simulink model "VELO1"  (R2019b)
settings: Solver=FixedStepAuto  StartTime=0.0  StopTime=t(end)  FixedStep=0.01  RelTol=1e-3
libraries: eeGeneralControl x26, dspstat3 x15, dspfdesign x11, sharedTrackingLibrary x2
(part 1 of 2)
settings Model: Creator=hosseini-a  LastModifiedBy=Ali
settings OptimizationCC: DefaultParameterBehavior=Inlined  EnhancedBackFolding=on  PassReuseOutputArgsAs=Individual arguments  ZeroExternalMemoryAtStartup=off  ZeroInternalMemoryAtStartup=off  OptimizeBlockOrder=speed  DifferentSizesBufferReuse=on  OptimizationCustomize=off  EfficientTunableParamExpr=on
settings DebuggingCC: ParameterTunabilityLossMsg=error
settings SFSimCC: MATLABDynamicMemAlloc=off
settings RTWCC: SystemTargetFile=ert.tlc  TemplateMakefile=ert_default_tmf  GenerateReport=on  IncludeHyperlinkInReport=on  LaunchReport=on  GenerateTraceInfo=on  GenerateTraceReport=on  GenerateTraceReportSl=on  GenerateTraceReportSf=on  GenerateTraceReportEml=on
settings CodeAppCC: ForceParamTrailComments=on  IgnoreCustomStorageClasses=off  OperatorAnnotations=on  SimulinkDataObjDesc=on  SFDataObjDesc=on  InsertBlockDesc=on
settings ERTTargetCC: TargetLangStandard=C99 (ISO)  GenerateSampleERTMain=on  InlinedParameterPlacement=NonHierarchical  ERTCustomFileTemplate=example_file_process.tlc

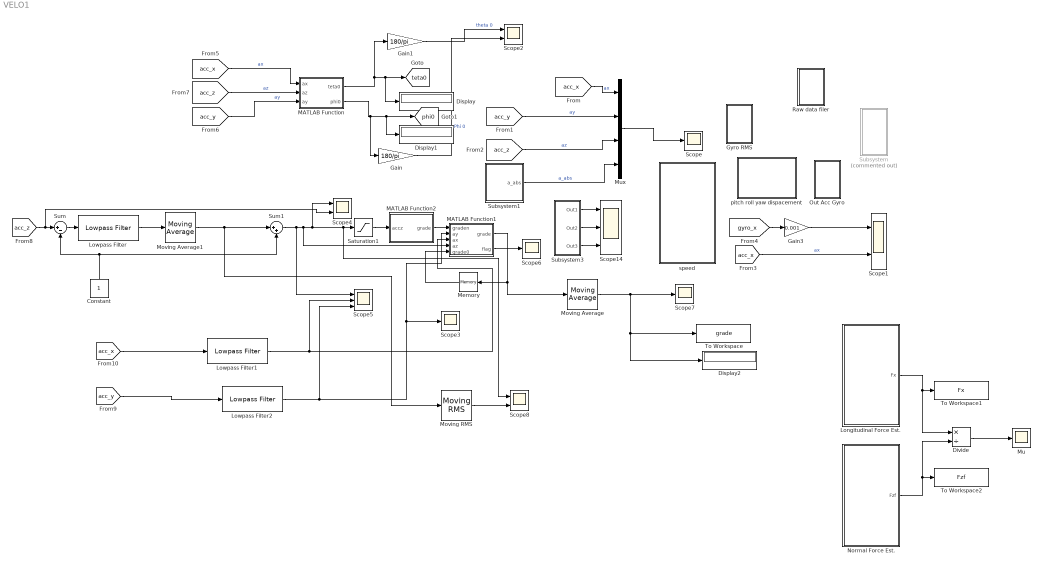
== system VELO1 ==
  Constant : Constant
  Display : Display
  Display1 : Display
  Display2 : Display
  Divide : Product  Inputs=*/
  Gain : Gain  Gain=180/pi
  Gain1 : Gain  Gain=180/pi
  Gain3 : Gain  Gain=0.001
  Gyro RMS : Subsystem
  Longitudinal Force Est. : Subsystem
  Lowpass Filter : dspfdesign/Lowpass Filter  FilterType=FIR  DesignForMinimumOrder=on  FilterOrder=50  PassbandFrequency=0.5  StopbandFrequency=1  PassbandRipple=0.05  StopbandAttenuation=20  InheritSampleRate=off  SampleRate=100  SimulateUsing=Interpreted execution  roundingMode=Floor  coeffsDataTypeStr=fixdt(1,16)
  Lowpass Filter1 : dspfdesign/Lowpass Filter  FilterType=FIR  DesignForMinimumOrder=on  FilterOrder=50  PassbandFrequency=1  StopbandFrequency=1.2  PassbandRipple=0.1  StopbandAttenuation=80  InheritSampleRate=off  SampleRate=100  SimulateUsing=Interpreted execution  roundingMode=Floor  coeffsDataTypeStr=fixdt(1,16)
  Lowpass Filter2 : dspfdesign/Lowpass Filter  FilterType=FIR  DesignForMinimumOrder=on  FilterOrder=50  PassbandFrequency=1  StopbandFrequency=1.2  PassbandRipple=0.1  StopbandAttenuation=80  InheritSampleRate=off  SampleRate=100  SimulateUsing=Interpreted execution  roundingMode=Floor  coeffsDataTypeStr=fixdt(1,16)
  MATLAB Function : MATLAB Function  TreatAsAtomicUnit=on
  MATLAB Function1 : MATLAB Function  TreatAsAtomicUnit=on
  MATLAB Function2 : MATLAB Function  TreatAsAtomicUnit=on
  Memory : Memory
  Moving Average : dspstat3/Moving Average  Method=Sliding window  ForgettingFactorPort=off  SpecifyWindowLength=on  WindowLength=100  ForgettingFactor=0.9  SimulateUsing=Code generation
  Moving Average1 : dspstat3/Moving Average  Method=Sliding window  ForgettingFactorPort=off  SpecifyWindowLength=on  WindowLength=100  ForgettingFactor=0.9  SimulateUsing=Code generation
  Moving RMS : dspstat3/Moving RMS  Method=Sliding window  ForgettingFactorPort=off  SpecifyWindowLength=on  WindowLength=100  ForgettingFactor=0.9  SimulateUsing=Code generation
      settings: SourceProductName=DSP System Toolbox  SourceProductBaseCode=DS
  Mu : Scope
  Mux : Mux
  Normal Force Est. : Subsystem
  Out Acc Gyro : Subsystem
  "Raw data filer " : Subsystem
  Saturation1 : Saturate  UpperLimit=1  LowerLimit=-0.981
  Scope{,3,6..7} (4 alike) : Scope
  Scope{1..2,4,8} (4 alike) : Scope  NumInputPorts=2
  Scope14 : Scope  NumInputPorts=3
  Scope5 : Scope  NumInputPorts=3
  Subsystem : Subsystem  Commented=on
  Subsystem1 : Subsystem
  Subsystem3 : Subsystem
  Sum : Sum  Inputs=|+-
  Sum1 : Sum  Inputs=|++
  To Workspace : ToWorkspace  VariableName=grade  SaveFormat=Timeseries  SampleTime=-1
  To Workspace1 : ToWorkspace  VariableName=Fx  SaveFormat=Timeseries  SampleTime=-1
  To Workspace2 : ToWorkspace  VariableName=Fzf  SaveFormat=Timeseries  SampleTime=-1
  pitch roll yaw dispacement : Subsystem
  speed : Subsystem
  tag scope: phi0=global, teta0=global
  wires:
  [acc_x] -> Mux/1  "ax"
  [acc_y] -> Mux/2  "ay"
  [acc_z] -> Mux/3  "az"
  Mux/1 -> Scope/1
  [gyro_x] -> Gain3/1
  [acc_x] -> Scope1/2  "ax"
  Gain3/1 -> Scope1/1
  Subsystem3/1(Out1) -> Scope14/1
  Subsystem3/2(Out2) -> Scope14/2
  Subsystem3/3(Out3) -> Scope14/3
  Subsystem1/1(a_abs) -> Mux/4  "a_abs"
  [acc_y] -> MATLAB Function/3(ay)  "ay"
  [acc_z] -> MATLAB Function/2(az)  "az"
  [acc_x] -> MATLAB Function/1(ax)  "ax"
  MATLAB Function/2(phi0) -> Gain/1, Display1/1, [phi0]
  MATLAB Function/1(teta0) -> Gain1/1, Display/1, [teta0]
  Gain1/1 -> Scope2/1  "theta 0"
  Gain/1 -> Scope2/2  "Phi 0"
  Saturation1/1 -> MATLAB Function2/1(accz)
  [acc_y] -> Lowpass Filter2/1
  Memory/1 -> MATLAB Function1/5(grade0)
  MATLAB Function2/1(grade) -> MATLAB Function1/1(graden)
  MATLAB Function1/1(grade) -> Moving Average/1, Memory/1
  [acc_x] -> Lowpass Filter1/1
  [acc_z] -> Scope4/2, Sum/1
  Sum/1 -> Lowpass Filter/1
  Lowpass Filter/1 -> Moving Average1/1
  Constant/1 -> Sum/2, Sum1/2
  Sum1/1 -> Scope5/1, MATLAB Function1/4(az), Scope4/1, Scope8/1, Saturation1/1
  Lowpass Filter1/1 -> Scope5/2, MATLAB Function1/3(ax)
  Lowpass Filter2/1 -> Scope5/3, MATLAB Function1/2(ay), Scope3/1
  MATLAB Function1/2(flag) -> Scope6/1
  Moving Average/1 -> Display2/1, To Workspace/1, Scope7/1
  Moving RMS/1 -> Scope8/2
  Moving Average1/1 -> Moving RMS/1, Sum1/1
  Longitudinal Force Est./1(Fx) -> To Workspace1/1, Divide/1
  Normal Force Est./1(Fzf) -> To Workspace2/1, Divide/2
  Divide/1 -> Mu/1

== system VELO1/Gyro RMS ==
  Moving RMS : dspstat3/Moving RMS  Method=Sliding window  ForgettingFactorPort=off  SpecifyWindowLength=on  WindowLength=50  ForgettingFactor=0.9  SimulateUsing=Code generation
      settings: SourceProductName=DSP System Toolbox  SourceProductBaseCode=DS
  Moving RMS1 : dspstat3/Moving RMS  Method=Sliding window  ForgettingFactorPort=off  SpecifyWindowLength=on  WindowLength=50  ForgettingFactor=0.9  SimulateUsing=Code generation
      settings: SourceProductName=DSP System Toolbox  SourceProductBaseCode=DS
  Moving RMS2 : dspstat3/Moving RMS  Method=Sliding window  ForgettingFactorPort=off  SpecifyWindowLength=on  WindowLength=50  ForgettingFactor=0.9  SimulateUsing=Code generation
      settings: SourceProductName=DSP System Toolbox  SourceProductBaseCode=DS
  Mux2 : Mux  Inputs=3
  Scope2 : Scope
  To Workspace2 : ToWorkspace  VariableName=rms_gyro  SaveFormat=Timeseries  SampleTime=-1
  wires:
  [gyro_z] -> Moving RMS1/1
  [gyro_y] -> Moving RMS2/1
  [gyro_x] -> Moving RMS/1
  Moving RMS/1 -> Mux2/1
  Mux2/1 -> Scope2/1, To Workspace2/1
  Moving RMS2/1 -> Mux2/2
  Moving RMS1/1 -> Mux2/3

== system VELO1/Longitudinal Force Est. ==
  Constant : Constant  Value=1500
  Constant1 : Constant  Value=1500
  MATLAB Function : MATLAB Function  TreatAsAtomicUnit=on
  MATLAB Function1 : MATLAB Function  TreatAsAtomicUnit=on
  Scope2 : Scope  NumInputPorts=2
  Fx : Outport
  wires:
  [acc_x] -> MATLAB Function/1(Ax)  "ax"
  [v_fuz] -> MATLAB Function/2(Vx)  "v_fuz"
  Constant/1 -> MATLAB Function/3(m)
  MATLAB Function1/1(Fx) -> Scope2/2  "Fx_w2"
  Constant1/1 -> MATLAB Function1/3(m)
  [V_w2] -> MATLAB Function1/2(Vx)  "ax"
  [acc_x] -> MATLAB Function1/1(Ax)  "ax"
  MATLAB Function/1(Fx) -> Fx/1, Scope2/1  "Fx_fuz"

== system VELO1/Normal Force Est. ==
  Constant : Constant  Value=1500
  Constant1 : Constant  Value=1500
  MATLAB Function : MATLAB Function  TreatAsAtomicUnit=on
  MATLAB Function1 : MATLAB Function  TreatAsAtomicUnit=on
  Scope2 : Scope  NumInputPorts=4
  Fzf : Outport
  wires:
  Constant/1 -> MATLAB Function/3(m)
  [v_fuz] -> MATLAB Function/2(Vx)  "v_fuz"
  [acc_x] -> MATLAB Function1/1(Ax)  "ax"
  [acc_x] -> MATLAB Function/1(Ax)  "ax"
  Constant1/1 -> MATLAB Function1/3(m)
  [V_w2] -> MATLAB Function1/2(Vx)  "ax"
  MATLAB Function1/2(Fzr) -> Scope2/4  "Fzr_w2"
  MATLAB Function/1(Fzf) -> Fzf/1, Scope2/1  "Fzf_fuz"
  MATLAB Function/2(Fzr) -> Scope2/2  "Fzr_fuz"
  MATLAB Function1/1(Fzf) -> Scope2/3  "Fzf_w2"

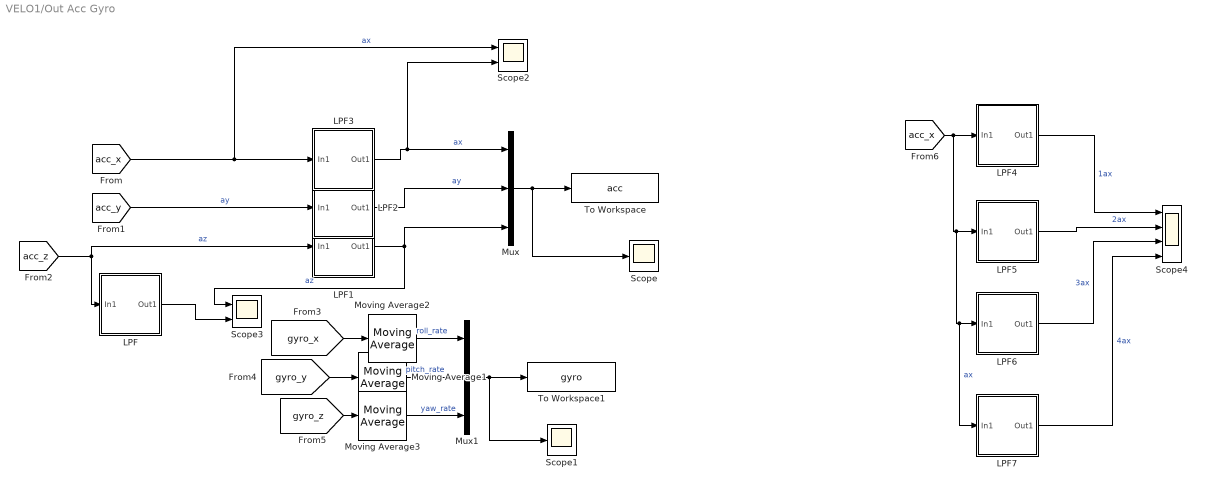
== system VELO1/Out Acc Gyro ==
  LPF : Subsystem
  LPF1 : Subsystem
  LPF2 : Subsystem
  LPF3 : Subsystem
  LPF4 : Subsystem
  LPF5 : Subsystem
  LPF6 : Subsystem
  LPF7 : Subsystem
  Moving Average1 : dspstat3/Moving Average  Method=Sliding window  ForgettingFactorPort=off  SpecifyWindowLength=on  WindowLength=200  ForgettingFactor=0.9  SimulateUsing=Code generation
  Moving Average2 : dspstat3/Moving Average  Method=Sliding window  ForgettingFactorPort=off  SpecifyWindowLength=on  WindowLength=200  ForgettingFactor=0.9  SimulateUsing=Code generation
  Moving Average3 : dspstat3/Moving Average  Method=Sliding window  ForgettingFactorPort=off  SpecifyWindowLength=on  WindowLength=200  ForgettingFactor=0.9  SimulateUsing=Code generation
  Mux : Mux  Inputs=3
  Mux1 : Mux  Inputs=3
  Scope : Scope
  Scope1 : Scope
  Scope2 : Scope  NumInputPorts=2
  Scope3 : Scope  NumInputPorts=2
  Scope4 : Scope  NumInputPorts=4
  To Workspace : ToWorkspace  VariableName=acc  SaveFormat=Timeseries  SampleTime=-1
  To Workspace1 : ToWorkspace  VariableName=gyro  SaveFormat=Timeseries  SampleTime=-1
  wires:
  [gyro_y] -> Moving Average1/1
  [gyro_x] -> Moving Average2/1
  [gyro_z] -> Moving Average3/1
  Mux1/1 -> To Workspace1/1, Scope1/1
  Moving Average1/1 -> Mux1/2  "pitch_rate"
  Moving Average2/1 -> Mux1/1  "roll_rate"
  Moving Average3/1 -> Mux1/3  "yaw_rate"
  [acc_z] -> LPF1/1(In1), LPF/1(In1)  "az"
  Mux/1 -> Scope/1, To Workspace/1
  [acc_x] -> Scope2/1, LPF3/1(In1)  "ax"
  [acc_y] -> LPF2/1(In1)  "ay"
  LPF1/1(Out1) -> Scope3/1, Mux/3  "az"
  LPF2/1(Out1) -> Mux/2  "ay"
  LPF3/1(Out1) -> Scope2/2, Mux/1  "ax"
  LPF/1(Out1) -> Scope3/2
  [acc_x] -> LPF7/1(In1), LPF6/1(In1), LPF5/1(In1), LPF4/1(In1)  "ax"
  LPF4/1(Out1) -> Scope4/1  "1ax"
  LPF5/1(Out1) -> Scope4/2  "2ax"
  LPF6/1(Out1) -> Scope4/3  "3ax"
  LPF7/1(Out1) -> Scope4/4  "4ax"

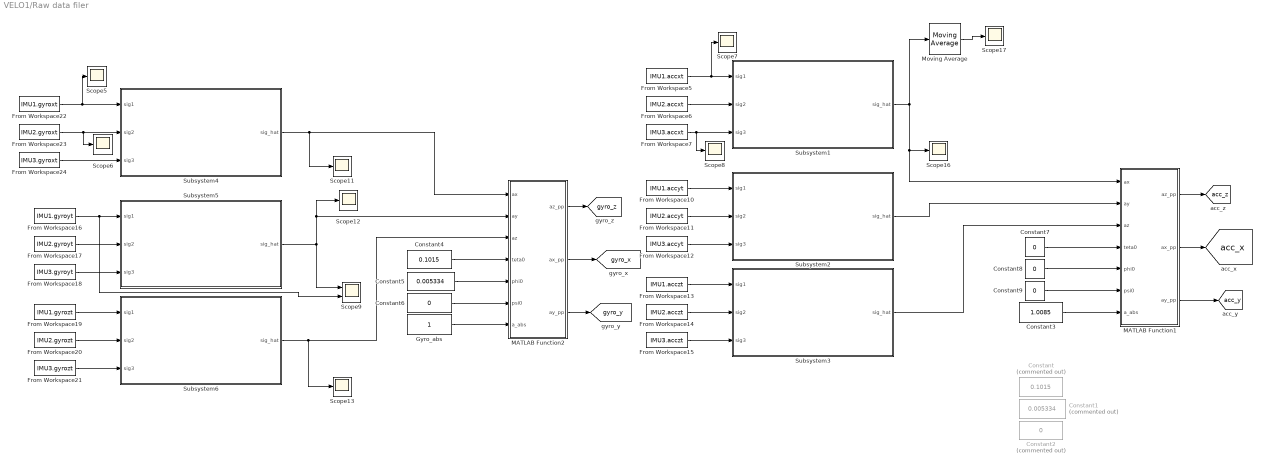
== system VELO1/Raw data filer  ==
  Constant : Constant  Commented=on  Value=0.1015
  Constant1 : Constant  Commented=on  Value=0.005334
  Constant2 : Constant  Commented=on  Value=0
  Constant3 : Constant  Value=1.0085
  Constant4 : Constant  Value=0.1015
  Constant5 : Constant  Value=0.005334
  Constant{6..9} (4 alike) : Constant  Value=0
  From Workspace10 : FromWorkspace  VariableName=IMU1.accyt  SampleTime=0
  From Workspace11 : FromWorkspace  VariableName=IMU2.accyt  SampleTime=0
  From Workspace12 : FromWorkspace  VariableName=IMU3.accyt  SampleTime=0
  From Workspace13 : FromWorkspace  VariableName=IMU1.acczt  SampleTime=0
  From Workspace14 : FromWorkspace  VariableName=IMU2.acczt  SampleTime=0
  From Workspace15 : FromWorkspace  VariableName=IMU3.acczt  SampleTime=0
  From Workspace16 : FromWorkspace  VariableName=IMU1.gyroyt  SampleTime=0
  From Workspace17 : FromWorkspace  VariableName=IMU2.gyroyt  SampleTime=0
  From Workspace18 : FromWorkspace  VariableName=IMU3.gyroyt  SampleTime=0
  From Workspace19 : FromWorkspace  VariableName=IMU1.gyrozt  SampleTime=0
  From Workspace20 : FromWorkspace  VariableName=IMU2.gyrozt  SampleTime=0
  From Workspace21 : FromWorkspace  VariableName=IMU3.gyrozt  SampleTime=0
  From Workspace22 : FromWorkspace  VariableName=IMU1.gyroxt  SampleTime=0
  From Workspace23 : FromWorkspace  VariableName=IMU2.gyroxt  SampleTime=0
  From Workspace24 : FromWorkspace  VariableName=IMU3.gyroxt  SampleTime=0
  From Workspace5 : FromWorkspace  VariableName=IMU1.accxt  SampleTime=0
  From Workspace6 : FromWorkspace  VariableName=IMU2.accxt  SampleTime=0
  From Workspace7 : FromWorkspace  VariableName=IMU3.accxt  SampleTime=0
  Gyro_abs : Constant
  MATLAB Function1 : MATLAB Function  TreatAsAtomicUnit=on
  MATLAB Function2 : MATLAB Function  TreatAsAtomicUnit=on
  Moving Average : dspstat3/Moving Average  Method=Sliding window  ForgettingFactorPort=off  SpecifyWindowLength=on  WindowLength=100  ForgettingFactor=0.9  SimulateUsing=Code generation
  Scope{5..8,11..13,16..17} (9 alike) : Scope
  Scope9 : Scope  NumInputPorts=2
  Subsystem1 : Subsystem
  Subsystem2 : Subsystem
  Subsystem3 : Subsystem
  Subsystem4 : Subsystem
  Subsystem5 : Subsystem
  Subsystem6 : Subsystem
  tag scope: acc_x=global, acc_y=global, acc_z=global, gyro_x=global, gyro_y=global, gyro_z=global
  wires:
  Subsystem6/1(sig_hat) -> MATLAB Function2/3(az), Scope13/1
  From Workspace20/1 -> Subsystem6/2(sig2)
  From Workspace15/1 -> Subsystem3/3(sig3)
  From Workspace13/1 -> Subsystem3/1(sig1)
  From Workspace7/1 -> Scope8/1, Subsystem1/3(sig3)
  From Workspace16/1 -> Scope9/2, Subsystem5/1(sig1)
  From Workspace11/1 -> Subsystem2/2(sig2)
  Subsystem3/1(sig_hat) -> MATLAB Function1/3(az)
  Subsystem1/1(sig_hat) -> MATLAB Function1/1(ax), Scope16/1, Moving Average/1
  From Workspace19/1 -> Subsystem6/1(sig1)
  From Workspace12/1 -> Subsystem2/3(sig3)
  From Workspace14/1 -> Subsystem3/2(sig2)
  From Workspace21/1 -> Subsystem6/3(sig3)
  From Workspace6/1 -> Subsystem1/2(sig2)
  From Workspace23/1 -> Scope6/1, Subsystem4/2(sig2)
  Subsystem4/1(sig_hat) -> MATLAB Function2/1(ax), Scope11/1
  Subsystem5/1(sig_hat) -> Scope12/1, MATLAB Function2/2(ay), Scope9/1
  From Workspace18/1 -> Subsystem5/3(sig3)
  From Workspace22/1 -> Scope5/1, Subsystem4/1(sig1)
  From Workspace10/1 -> Subsystem2/1(sig1)
  From Workspace5/1 -> Scope7/1, Subsystem1/1(sig1)
  From Workspace24/1 -> Subsystem4/3(sig3)
  From Workspace17/1 -> Subsystem5/2(sig2)
  Moving Average/1 -> Scope17/1
  Subsystem2/1(sig_hat) -> MATLAB Function1/2(ay)
  Constant3/1 -> MATLAB Function1/7(a_abs)
  Constant7/1 -> MATLAB Function1/4(teta0)
  Constant8/1 -> MATLAB Function1/5(phi0)
  Constant9/1 -> MATLAB Function1/6(psi0)
  Constant5/1 -> MATLAB Function2/5(phi0)
  Constant4/1 -> MATLAB Function2/4(teta0)
  Constant6/1 -> MATLAB Function2/6(psi0)
  Gyro_abs/1 -> MATLAB Function2/7(a_abs)
  MATLAB Function2/2(ax_pp) -> [gyro_x]
  MATLAB Function2/3(ay_pp) -> [gyro_y]
  MATLAB Function2/1(az_pp) -> [gyro_z]
  MATLAB Function1/1(az_pp) -> [acc_z]
  MATLAB Function1/2(ax_pp) -> [acc_x]
  MATLAB Function1/3(ay_pp) -> [acc_y]

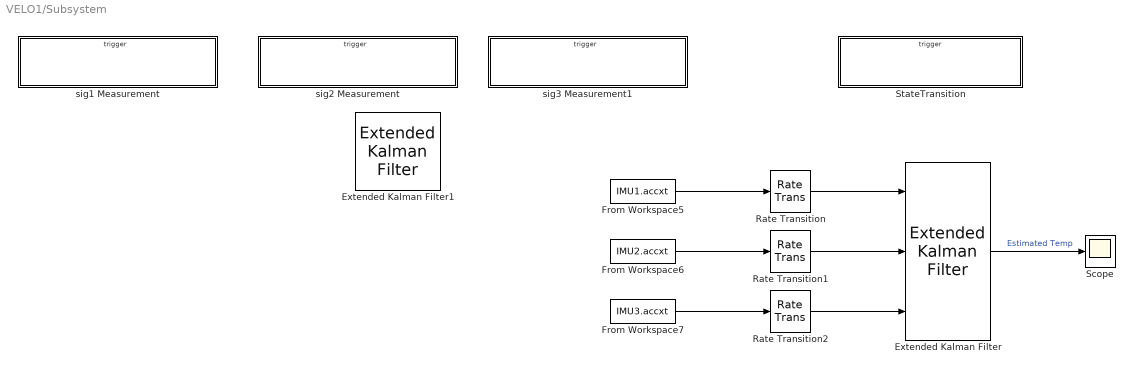
== system VELO1/Subsystem ==
  Extended Kalman Filter : sharedTrackingLibrary/Extended Kalman Filter  StateTransitionFcn=stateTransitionFcn  HasStateTransitionJacobianFcn=off  HasAdditiveProcessNoise=Nonadditive  ProcessNoise=0.5  HasTimeVaryingProcessNoise=off  HasStateTransitionFcnExtraArgument=0  InitialState=0  InitialStateCovariance=1  MeasurementFcn1=sig1MeasurementFcn  HasMeasurementJacobianFcn1=off  HasMeasurementEnablePort1=off  HasAdditiveMeasurementNoise1=Nonadditive  MeasurementNoise1=0.2  HasTimeVaryingMeasurementNoise1=off  HasMeasurementFcnExtraArgument1=0  MeasurementFcn2=sig2MeasurementFcn  HasMeasurementJacobianFcn2=off  HasMeasurementEnablePort2=off  HasAdditiveMeasurementNoise2=Nonadditive  MeasurementNoise2=0.2  HasTimeVaryingMeasurementNoise2=off  HasMeasurementFcnExtraArgument2=0  MeasurementFcn3=sig3MeasurementFcn  HasMeasurementJacobianFcn3=off  HasMeasurementEnablePort3=off  HasAdditiveMeasurementNoise3=Nonadditive  MeasurementNoise3=1  HasTimeVaryingMeasurementNoise3=off  HasMeasurementFcnExtraArgument3=0  MeasurementFcn4=myMeasurementFcn  HasMeasurementJacobianFcn4=off  HasMeasurementEnablePort4=off  HasAdditiveMeasurementNoise4=Additive  MeasurementNoise4=1  HasTimeVaryingMeasurementNoise4=off  HasMeasurementFcnExtraArgument4=0  MeasurementFcn5=myMeasurementFcn  HasMeasurementJacobianFcn5=off  HasMeasurementEnablePort5=off  HasAdditiveMeasurementNoise5=Additive  MeasurementNoise5=1  HasTimeVaryingMeasurementNoise5=off  HasMeasurementFcnExtraArgument5=0  EnableMultirate=off  StateTransitionFcnSampleTime=1  MeasurementFcn1SampleTime=1  MeasurementFcn2SampleTime=1  MeasurementFcn3SampleTime=1  MeasurementFcn4SampleTime=1  MeasurementFcn5SampleTime=1  UseCurrentEstimator=on  OutputStateCovariance=off  DataType=double  SampleTime=0.01  NumberOfMeasurements=3
      settings: SourceProductName=Control System Toolbox  SourceProductBaseCode=CT
  Extended Kalman Filter1 : sharedTrackingLibrary/Extended Kalman Filter  StateTransitionFcn=myStateTransitionFcn  HasStateTransitionJacobianFcn=off  HasAdditiveProcessNoise=Additive  ProcessNoise=1  HasTimeVaryingProcessNoise=off  HasStateTransitionFcnExtraArgument=0  InitialState=0  InitialStateCovariance=1  MeasurementFcn1=myMeasurementFcn  HasMeasurementJacobianFcn1=off  HasMeasurementEnablePort1=off  HasAdditiveMeasurementNoise1=Additive  MeasurementNoise1=1  HasTimeVaryingMeasurementNoise1=off  HasMeasurementFcnExtraArgument1=0  MeasurementFcn2=myMeasurementFcn  HasMeasurementJacobianFcn2=off  HasMeasurementEnablePort2=off  HasAdditiveMeasurementNoise2=Additive  MeasurementNoise2=1  HasTimeVaryingMeasurementNoise2=off  HasMeasurementFcnExtraArgument2=0  MeasurementFcn3=myMeasurementFcn  HasMeasurementJacobianFcn3=off  HasMeasurementEnablePort3=off  HasAdditiveMeasurementNoise3=Additive  MeasurementNoise3=1  HasTimeVaryingMeasurementNoise3=off  HasMeasurementFcnExtraArgument3=0  MeasurementFcn4=myMeasurementFcn  HasMeasurementJacobianFcn4=off  HasMeasurementEnablePort4=off  HasAdditiveMeasurementNoise4=Additive  MeasurementNoise4=1  HasTimeVaryingMeasurementNoise4=off  HasMeasurementFcnExtraArgument4=0  MeasurementFcn5=myMeasurementFcn  HasMeasurementJacobianFcn5=off  HasMeasurementEnablePort5=off  HasAdditiveMeasurementNoise5=Additive  MeasurementNoise5=1  HasTimeVaryingMeasurementNoise5=off  HasMeasurementFcnExtraArgument5=0  EnableMultirate=off  StateTransitionFcnSampleTime=1  MeasurementFcn1SampleTime=1  MeasurementFcn2SampleTime=1  MeasurementFcn3SampleTime=1  MeasurementFcn4SampleTime=1  MeasurementFcn5SampleTime=1  UseCurrentEstimator=on  OutputStateCovariance=off  DataType=double  SampleTime=1  NumberOfMeasurements=1
      settings: SourceProductName=Automated Driving Toolbox  SourceProductBaseCode=DR
  From Workspace5 : FromWorkspace  VariableName=IMU1.accxt  SampleTime=0
  From Workspace6 : FromWorkspace  VariableName=IMU2.accxt  SampleTime=0
  From Workspace7 : FromWorkspace  VariableName=IMU3.accxt  SampleTime=0
  Rate Transition : RateTransition
  Rate Transition1 : RateTransition
  Rate Transition2 : RateTransition
  Scope : Scope
  StateTransition : Subsystem  TreatAsAtomicUnit=on
  sig1 Measurement : Subsystem  TreatAsAtomicUnit=on
  sig2 Measurement : Subsystem  TreatAsAtomicUnit=on
  sig3 Measurement1 : Subsystem  TreatAsAtomicUnit=on
  wires:
  Extended Kalman Filter/1 -> Scope/1  "Estimated Temp"
  Rate Transition1/1 -> Extended Kalman Filter/2
  Rate Transition/1 -> Extended Kalman Filter/1
  Rate Transition2/1 -> Extended Kalman Filter/3
  From Workspace5/1 -> Rate Transition/1
  From Workspace6/1 -> Rate Transition1/1
  From Workspace7/1 -> Rate Transition2/1

== system VELO1/Subsystem1 ==
  MATLAB Function : MATLAB Function  TreatAsAtomicUnit=on
  a_abs : Outport
  wires:
  [acc_y] -> MATLAB Function/2(ay)  "ay"
  [acc_x] -> MATLAB Function/1(ax)  "ax"
  [acc_z] -> MATLAB Function/3(az)  "az"
  MATLAB Function/1(a) -> a_abs/1  "a_abs"

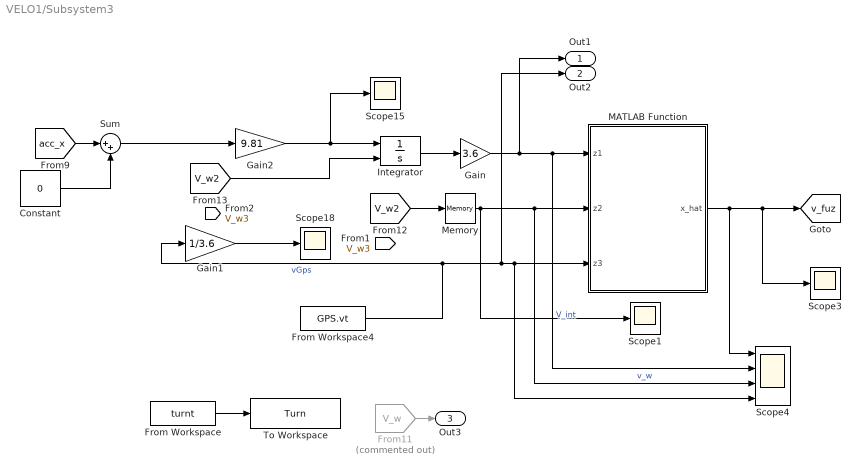
== system VELO1/Subsystem3 ==
  Constant : Constant  Value=0
  From Workspace : FromWorkspace  VariableName=turnt  SampleTime=0
  From Workspace4 : FromWorkspace  VariableName=GPS.vt  SampleTime=0
  From11 : From  Commented=on  GotoTag=V_w  TagVisibility=global
  Gain : Gain  Gain=3.6
  Gain1 : Gain  Gain=1/3.6
  Gain2 : Gain  Gain=9.81
  Integrator : Integrator  InitialConditionSource=external  ContinuousStateAttributes='Velocity'
  MATLAB Function : MATLAB Function  TreatAsAtomicUnit=on
  Memory : Memory
  Scope{1,3,15,18} (4 alike) : Scope
  Scope4 : Scope  NumInputPorts=4
  Sum : Sum  Inputs=|++
  To Workspace : ToWorkspace  VariableName=Turn  SaveFormat=Timeseries  SampleTime=-1
  Out1 : Outport
  Out2 : Outport  Port=2
  Out3 : Outport  Port=3
  tag scope: v_fuz=global
  wires:
  [V_w2] -> Memory/1
  Memory/1 -> Scope1/1, Scope4/3, MATLAB Function/2(z2)  "v_w"
  Gain/1 -> Out1/1, Scope4/2, MATLAB Function/1(z1)  "V_int"
  Constant/1 -> Sum/2
  MATLAB Function/1(x_hat) -> Scope3/1, [v_fuz], Scope4/1
  Gain2/1 -> Scope15/1, Integrator/1
  [acc_x] -> Sum/1
  Gain1/1 -> Scope18/1
  Sum/1 -> Gain2/1
  From Workspace4/1 -> Gain1/1, Out2/1, Scope4/4, MATLAB Function/3(z3)  "vGps"
  [V_w2] -> Integrator/2
  Integrator/1 -> Gain/1
  From11/1 -> Out3/1
  From Workspace/1 -> To Workspace/1

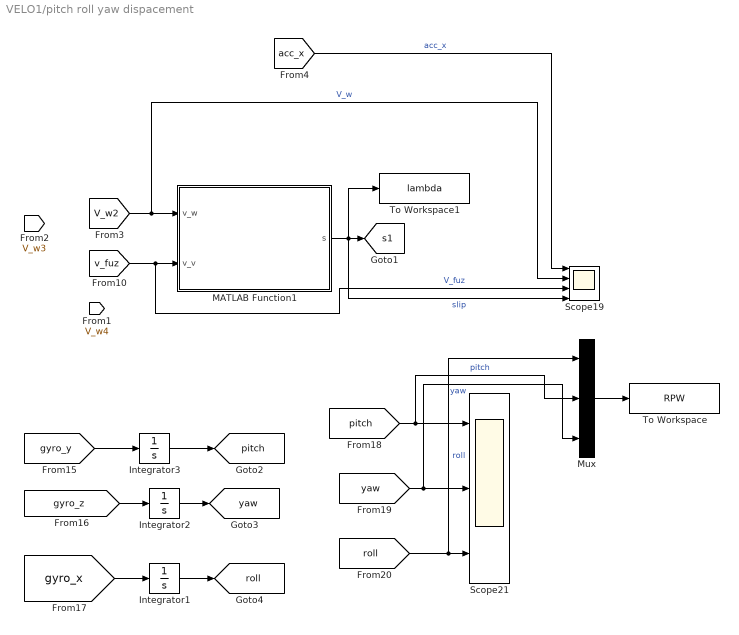
== system VELO1/pitch roll yaw dispacement ==
  Integrator1 : Integrator
  Integrator2 : Integrator
  Integrator3 : Integrator
  MATLAB Function1 : MATLAB Function  TreatAsAtomicUnit=on
  Mux : Mux  Inputs=3
  Scope19 : Scope  NumInputPorts=4
  Scope21 : Scope  NumInputPorts=3
  To Workspace : ToWorkspace  VariableName=RPW  SaveFormat=Timeseries  SampleTime=-1
  To Workspace1 : ToWorkspace  VariableName=lambda  SaveFormat=Timeseries  SampleTime=-1
  tag scope: pitch=global, roll=global, s1=global, yaw=global
  wires:
  [gyro_x] -> Integrator1/1
  [v_fuz] -> Scope19/3, MATLAB Function1/2(v_v)  "V_fuz"
  [gyro_y] -> Integrator3/1
  Integrator1/1 -> [roll]
  [V_w2] -> Scope19/2, MATLAB Function1/1(v_w)  "V_w"
  [roll] -> Mux/1, Scope21/3  "roll"
  Integrator3/1 -> [pitch]
  MATLAB Function1/1(s) -> Scope19/4, To Workspace1/1, [s1]  "slip"
  [pitch] -> Mux/2, Scope21/1  "pitch"
  [yaw] -> Mux/3, Scope21/2  "yaw"
  Integrator2/1 -> [yaw]
  [gyro_z] -> Integrator2/1
  Mux/1 -> To Workspace/1
  [acc_x] -> Scope19/1  "acc_x"

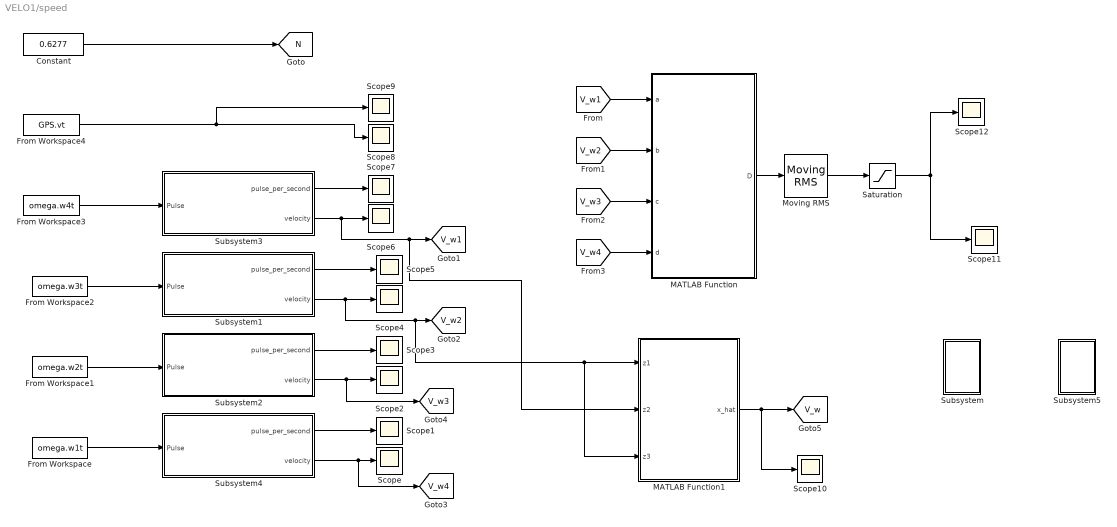
== system VELO1/speed ==
  Constant : Constant  Value=0.6277
  From Workspace : FromWorkspace  VariableName=omega.w1t  SampleTime=0
  From Workspace1 : FromWorkspace  VariableName=omega.w2t  SampleTime=0
  From Workspace2 : FromWorkspace  VariableName=omega.w3t  SampleTime=0
  From Workspace3 : FromWorkspace  VariableName=omega.w4t  SampleTime=0
  From Workspace4 : FromWorkspace  VariableName=GPS.vt  SampleTime=0
  MATLAB Function : MATLAB Function  TreatAsAtomicUnit=on
  MATLAB Function1 : MATLAB Function  TreatAsAtomicUnit=on
  Moving RMS : dspstat3/Moving RMS  Method=Sliding window  ForgettingFactorPort=off  SpecifyWindowLength=on  WindowLength=100  ForgettingFactor=0.9  SimulateUsing=Code generation
      settings: SourceProductName=DSP System Toolbox  SourceProductBaseCode=DS
  Saturation : Saturate  UpperLimit=1.05  LowerLimit=0.95
  Scope{,1..12} (13 alike) : Scope
  Subsystem : Subsystem
  Subsystem1 : Subsystem
  Subsystem2 : Subsystem
  Subsystem3 : Subsystem
  Subsystem4 : Subsystem
  Subsystem5 : Subsystem
  tag scope: N=global, V_w1=global, V_w2=global, V_w3=global, V_w4=global, V_w=global
  wires:
  From Workspace3/1 -> Subsystem3/1(Pulse)
  From Workspace1/1 -> Subsystem2/1(Pulse)
  Saturation/1 -> Scope12/1, Scope11/1
  [V_w1] -> MATLAB Function/1(a)
  Subsystem4/2(velocity) -> [V_w4], Scope/1
  [V_w2] -> MATLAB Function/2(b)
  From Workspace/1 -> Subsystem4/1(Pulse)
  Subsystem4/1(pulse_per_second) -> Scope1/1
  Subsystem1/1(pulse_per_second) -> Scope5/1
  Subsystem1/2(velocity) -> MATLAB Function1/3(z3), MATLAB Function1/1(z1), [V_w2], Scope4/1
  From Workspace2/1 -> Subsystem1/1(Pulse)
  From Workspace4/1 -> Scope8/1, Scope9/1
  Constant/1 -> [N]
  Subsystem3/2(velocity) -> MATLAB Function1/2(z2), [V_w1], Scope6/1
  Moving RMS/1 -> Saturation/1
  [V_w4] -> MATLAB Function/4(d)
  [V_w3] -> MATLAB Function/3(c)
  Subsystem2/1(pulse_per_second) -> Scope3/1
  Subsystem2/2(velocity) -> [V_w3], Scope2/1
  MATLAB Function/1(D) -> Moving RMS/1
  Subsystem3/1(pulse_per_second) -> Scope7/1
  MATLAB Function1/1(x_hat) -> Scope10/1, [V_w]

== system VELO1/Out Acc Gyro/LPF ==
  In1 : Inport
  Constant : Constant
  Lowpass Filter : dspfdesign/Lowpass Filter  FilterType=FIR  DesignForMinimumOrder=on  FilterOrder=50  PassbandFrequency=10  StopbandFrequency=11  PassbandRipple=0.1  StopbandAttenuation=30  InheritSampleRate=off  SampleRate=100  SimulateUsing=Interpreted execution  roundingMode=Floor  coeffsDataTypeStr=fixdt(1,16)
  Sum : Sum  Inputs=|+-
  Sum1 : Sum  Inputs=|++
  Out1 : Outport
  wires:
  In1/1 -> Sum/1
  Lowpass Filter/1 -> Sum1/1
  Constant/1 -> Sum/2, Sum1/2
  Sum/1 -> Lowpass Filter/1
  Sum1/1 -> Out1/1

== system VELO1/Out Acc Gyro/LPF1 ==
  In1 : Inport
  Constant : Constant
  Lowpass Filter : dspfdesign/Lowpass Filter  FilterType=FIR  DesignForMinimumOrder=on  FilterOrder=50  PassbandFrequency=5  StopbandFrequency=10  PassbandRipple=0.1  StopbandAttenuation=30  InheritSampleRate=off  SampleRate=100  SimulateUsing=Interpreted execution  roundingMode=Floor  coeffsDataTypeStr=fixdt(1,16)
  Sum : Sum  Inputs=|+-
  Sum1 : Sum  Inputs=|++
  Out1 : Outport
  wires:
  Sum1/1 -> Out1/1
  Sum/1 -> Lowpass Filter/1
  Constant/1 -> Sum1/2, Sum/2
  Lowpass Filter/1 -> Sum1/1
  In1/1 -> Sum/1

== system VELO1/Out Acc Gyro/LPF2 ==
  In1 : Inport
  Constant : Constant  Value=0
  Lowpass Filter : dspfdesign/Lowpass Filter  FilterType=FIR  DesignForMinimumOrder=on  FilterOrder=50  PassbandFrequency=5  StopbandFrequency=10  PassbandRipple=0.1  StopbandAttenuation=30  InheritSampleRate=off  SampleRate=100  SimulateUsing=Interpreted execution  roundingMode=Floor  coeffsDataTypeStr=fixdt(1,16)
  Sum : Sum  Inputs=|+-
  Sum1 : Sum  Inputs=|++
  Out1 : Outport
  wires:
  In1/1 -> Sum/1
  Lowpass Filter/1 -> Sum1/1
  Constant/1 -> Sum/2, Sum1/2
  Sum/1 -> Lowpass Filter/1
  Sum1/1 -> Out1/1

== system VELO1/Out Acc Gyro/LPF3 ==
  In1 : Inport
  Constant : Constant  Value=0
  Lowpass Filter : dspfdesign/Lowpass Filter  FilterType=FIR  DesignForMinimumOrder=on  FilterOrder=50  PassbandFrequency=5  StopbandFrequency=10  PassbandRipple=0.1  StopbandAttenuation=30  InheritSampleRate=off  SampleRate=100  SimulateUsing=Interpreted execution  roundingMode=Floor  coeffsDataTypeStr=fixdt(1,16)
  Sum : Sum  Inputs=|+-
  Sum1 : Sum  Inputs=|++
  Out1 : Outport
  wires:
  Sum1/1 -> Out1/1
  Sum/1 -> Lowpass Filter/1
  Constant/1 -> Sum1/2, Sum/2
  Lowpass Filter/1 -> Sum1/1
  In1/1 -> Sum/1

== system VELO1/Out Acc Gyro/LPF4 ==
  In1 : Inport
  Constant : Constant  Value=0
  Lowpass Filter : dspfdesign/Lowpass Filter  FilterType=FIR  DesignForMinimumOrder=on  FilterOrder=50  PassbandFrequency=5  StopbandFrequency=10  PassbandRipple=0.1  StopbandAttenuation=80  InheritSampleRate=off  SampleRate=100  SimulateUsing=Interpreted execution  roundingMode=Floor  coeffsDataTypeStr=fixdt(1,16)
  Sum : Sum  Inputs=|+-
  Sum1 : Sum  Inputs=|++
  Out1 : Outport
  wires:
  In1/1 -> Sum/1
  Lowpass Filter/1 -> Sum1/1
  Constant/1 -> Sum/2, Sum1/2
  Sum/1 -> Lowpass Filter/1
  Sum1/1 -> Out1/1

== system VELO1/Out Acc Gyro/LPF5 ==
  In1 : Inport
  Constant : Constant  Value=0
  Lowpass Filter : dspfdesign/Lowpass Filter  FilterType=FIR  DesignForMinimumOrder=on  FilterOrder=50  PassbandFrequency=5  StopbandFrequency=10  PassbandRipple=0.05  StopbandAttenuation=80  InheritSampleRate=off  SampleRate=100  SimulateUsing=Interpreted execution  roundingMode=Floor  coeffsDataTypeStr=fixdt(1,16)
  Sum : Sum  Inputs=|+-
  Sum1 : Sum  Inputs=|++
  Out1 : Outport
  wires:
  Sum1/1 -> Out1/1
  Sum/1 -> Lowpass Filter/1
  Constant/1 -> Sum1/2, Sum/2
  Lowpass Filter/1 -> Sum1/1
  In1/1 -> Sum/1

== system VELO1/Out Acc Gyro/LPF6 ==
  In1 : Inport
  Constant : Constant  Value=0
  Lowpass Filter : dspfdesign/Lowpass Filter  FilterType=FIR  DesignForMinimumOrder=on  FilterOrder=50  PassbandFrequency=5  StopbandFrequency=10  PassbandRipple=0.1  StopbandAttenuation=20  InheritSampleRate=off  SampleRate=100  SimulateUsing=Interpreted execution  roundingMode=Floor  coeffsDataTypeStr=fixdt(1,16)
  Sum : Sum  Inputs=|+-
  Sum1 : Sum  Inputs=|++
  Out1 : Outport
  wires:
  In1/1 -> Sum/1
  Lowpass Filter/1 -> Sum1/1
  Constant/1 -> Sum/2, Sum1/2
  Sum/1 -> Lowpass Filter/1
  Sum1/1 -> Out1/1

== system VELO1/Out Acc Gyro/LPF7 ==
  In1 : Inport
  Constant : Constant  Value=0
  Lowpass Filter : dspfdesign/Lowpass Filter  FilterType=IIR  DesignForMinimumOrder=on  FilterOrder=50  PassbandFrequency=5  StopbandFrequency=10  PassbandRipple=0.1  StopbandAttenuation=5  InheritSampleRate=off  SampleRate=100  SimulateUsing=Interpreted execution  roundingMode=Floor  coeffsDataTypeStr=fixdt(1,16)
  Sum : Sum  Inputs=|+-
  Sum1 : Sum  Inputs=|++
  Out1 : Outport
  wires:
  Sum1/1 -> Out1/1
  Sum/1 -> Lowpass Filter/1
  Constant/1 -> Sum1/2, Sum/2
  Lowpass Filter/1 -> Sum1/1
  In1/1 -> Sum/1

== system VELO1/Raw data filer /Subsystem1 ==
  sig1 : Inport
  sig2 : Inport  Port=2
  sig3 : Inport  Port=3
  Low-Pass Filter (Discrete or Continuous) : eeGeneralControl/Low-Pass Filter (Discrete or Continuous)  K=1  T=0.1  B=inf  A=-inf  Ts=-1
      settings: SourceProductName=Simscape Electrical
  Low-Pass Filter (Discrete or Continuous)1 : eeGeneralControl/Low-Pass Filter (Discrete or Continuous)  K=1  T=0.1  B=inf  A=-inf  Ts=-1
      settings: SourceProductName=Simscape Electrical
  Low-Pass Filter (Discrete or Continuous)2 : eeGeneralControl/Low-Pass Filter (Discrete or Continuous)  K=1  T=0.1  B=inf  A=-inf  Ts=-1
      settings: SourceProductName=Simscape Electrical
  MATLAB Function : MATLAB Function  TreatAsAtomicUnit=on
  sig_hat : Outport
  wires:
  Low-Pass Filter (Discrete or Continuous)1/1 -> MATLAB Function/3(z3)
  Low-Pass Filter (Discrete or Continuous)2/1 -> MATLAB Function/1(z1)
  sig2/1 -> Low-Pass Filter (Discrete or Continuous)/1
  sig1/1 -> Low-Pass Filter (Discrete or Continuous)2/1
  Low-Pass Filter (Discrete or Continuous)/1 -> MATLAB Function/2(z2)
  MATLAB Function/1(x_hat) -> sig_hat/1
  sig3/1 -> Low-Pass Filter (Discrete or Continuous)1/1

== system VELO1/Raw data filer /Subsystem2 ==
  sig1 : Inport
  sig2 : Inport  Port=2
  sig3 : Inport  Port=3
  Low-Pass Filter (Discrete or Continuous) : eeGeneralControl/Low-Pass Filter (Discrete or Continuous)  K=1  T=0.1  B=inf  A=-inf  Ts=-1
      settings: SourceProductName=Simscape Electrical
  Low-Pass Filter (Discrete or Continuous)1 : eeGeneralControl/Low-Pass Filter (Discrete or Continuous)  K=1  T=0.1  B=inf  A=-inf  Ts=-1
      settings: SourceProductName=Simscape Electrical
  Low-Pass Filter (Discrete or Continuous)2 : eeGeneralControl/Low-Pass Filter (Discrete or Continuous)  K=1  T=0.1  B=inf  A=-inf  Ts=-1
      settings: SourceProductName=Simscape Electrical
  MATLAB Function : MATLAB Function  TreatAsAtomicUnit=on
  sig_hat : Outport
  wires:
  sig3/1 -> Low-Pass Filter (Discrete or Continuous)1/1
  MATLAB Function/1(x_hat) -> sig_hat/1
  Low-Pass Filter (Discrete or Continuous)/1 -> MATLAB Function/2(z2)
  sig1/1 -> Low-Pass Filter (Discrete or Continuous)2/1
  sig2/1 -> Low-Pass Filter (Discrete or Continuous)/1
  Low-Pass Filter (Discrete or Continuous)2/1 -> MATLAB Function/1(z1)
  Low-Pass Filter (Discrete or Continuous)1/1 -> MATLAB Function/3(z3)

== system VELO1/Raw data filer /Subsystem3 ==
  sig1 : Inport
  sig2 : Inport  Port=2
  sig3 : Inport  Port=3
  Low-Pass Filter (Discrete or Continuous) : eeGeneralControl/Low-Pass Filter (Discrete or Continuous)  K=1  T=0.1  B=inf  A=-inf  Ts=-1
      settings: SourceProductName=Simscape Electrical
  Low-Pass Filter (Discrete or Continuous)1 : eeGeneralControl/Low-Pass Filter (Discrete or Continuous)  K=1  T=0.1  B=inf  A=-inf  Ts=-1
      settings: SourceProductName=Simscape Electrical
  Low-Pass Filter (Discrete or Continuous)2 : eeGeneralControl/Low-Pass Filter (Discrete or Continuous)  K=1  T=0.1  B=inf  A=-inf  Ts=-1
      settings: SourceProductName=Simscape Electrical
  MATLAB Function : MATLAB Function  TreatAsAtomicUnit=on
  sig_hat : Outport
  wires:
  Low-Pass Filter (Discrete or Continuous)1/1 -> MATLAB Function/3(z3)
  Low-Pass Filter (Discrete or Continuous)2/1 -> MATLAB Function/1(z1)
  sig2/1 -> Low-Pass Filter (Discrete or Continuous)/1
  sig1/1 -> Low-Pass Filter (Discrete or Continuous)2/1
  Low-Pass Filter (Discrete or Continuous)/1 -> MATLAB Function/2(z2)
  MATLAB Function/1(x_hat) -> sig_hat/1
  sig3/1 -> Low-Pass Filter (Discrete or Continuous)1/1

== system VELO1/Raw data filer /Subsystem4 ==
  sig1 : Inport
  sig2 : Inport  Port=2
  sig3 : Inport  Port=3
  Low-Pass Filter (Discrete or Continuous) : eeGeneralControl/Low-Pass Filter (Discrete or Continuous)  K=1  T=0.1  B=inf  A=-inf  Ts=-1
      settings: SourceProductName=Simscape Electrical
  Low-Pass Filter (Discrete or Continuous)1 : eeGeneralControl/Low-Pass Filter (Discrete or Continuous)  K=1  T=0.1  B=inf  A=-inf  Ts=-1
      settings: SourceProductName=Simscape Electrical
  Low-Pass Filter (Discrete or Continuous)2 : eeGeneralControl/Low-Pass Filter (Discrete or Continuous)  K=1  T=0.1  B=inf  A=-inf  Ts=-1
      settings: SourceProductName=Simscape Electrical
  MATLAB Function : MATLAB Function  TreatAsAtomicUnit=on
  sig_hat : Outport
  wires:
  sig3/1 -> Low-Pass Filter (Discrete or Continuous)1/1
  MATLAB Function/1(x_hat) -> sig_hat/1
  Low-Pass Filter (Discrete or Continuous)/1 -> MATLAB Function/2(z2)
  sig1/1 -> Low-Pass Filter (Discrete or Continuous)2/1
  sig2/1 -> Low-Pass Filter (Discrete or Continuous)/1
  Low-Pass Filter (Discrete or Continuous)2/1 -> MATLAB Function/1(z1)
  Low-Pass Filter (Discrete or Continuous)1/1 -> MATLAB Function/3(z3)

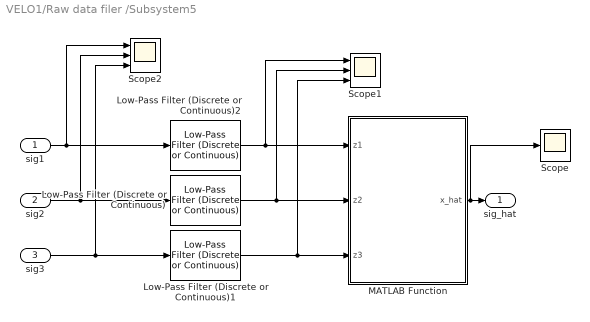
== system VELO1/Raw data filer /Subsystem5 ==
  sig1 : Inport
  sig2 : Inport  Port=2
  sig3 : Inport  Port=3
  Low-Pass Filter (Discrete or Continuous) : eeGeneralControl/Low-Pass Filter (Discrete or Continuous)  K=1  T=0.1  B=inf  A=-inf  Ts=-1
      settings: SourceProductName=Simscape Electrical
  Low-Pass Filter (Discrete or Continuous)1 : eeGeneralControl/Low-Pass Filter (Discrete or Continuous)  K=1  T=0.1  B=inf  A=-inf  Ts=-1
      settings: SourceProductName=Simscape Electrical
  Low-Pass Filter (Discrete or Continuous)2 : eeGeneralControl/Low-Pass Filter (Discrete or Continuous)  K=1  T=0.1  B=inf  A=-inf  Ts=-1
      settings: SourceProductName=Simscape Electrical
  MATLAB Function : MATLAB Function  TreatAsAtomicUnit=on
  Scope : Scope
  Scope1 : Scope  NumInputPorts=3
  Scope2 : Scope  NumInputPorts=3
  sig_hat : Outport
  wires:
  Low-Pass Filter (Discrete or Continuous)1/1 -> Scope1/3, MATLAB Function/3(z3)
  Low-Pass Filter (Discrete or Continuous)2/1 -> Scope1/1, MATLAB Function/1(z1)
  sig2/1 -> Scope2/2, Low-Pass Filter (Discrete or Continuous)/1
  sig1/1 -> Scope2/1, Low-Pass Filter (Discrete or Continuous)2/1
  Low-Pass Filter (Discrete or Continuous)/1 -> Scope1/2, MATLAB Function/2(z2)
  sig3/1 -> Scope2/3, Low-Pass Filter (Discrete or Continuous)1/1
  MATLAB Function/1(x_hat) -> Scope/1, sig_hat/1

== system VELO1/Raw data filer /Subsystem6 ==
  sig1 : Inport
  sig2 : Inport  Port=2
  sig3 : Inport  Port=3
  Low-Pass Filter (Discrete or Continuous) : eeGeneralControl/Low-Pass Filter (Discrete or Continuous)  K=1  T=0.1  B=inf  A=-inf  Ts=-1
      settings: SourceProductName=Simscape Electrical
  Low-Pass Filter (Discrete or Continuous)1 : eeGeneralControl/Low-Pass Filter (Discrete or Continuous)  K=1  T=0.1  B=inf  A=-inf  Ts=-1
      settings: SourceProductName=Simscape Electrical
  Low-Pass Filter (Discrete or Continuous)2 : eeGeneralControl/Low-Pass Filter (Discrete or Continuous)  K=1  T=0.1  B=inf  A=-inf  Ts=-1
      settings: SourceProductName=Simscape Electrical
  MATLAB Function : MATLAB Function  TreatAsAtomicUnit=on
  sig_hat : Outport
  wires:
  sig3/1 -> Low-Pass Filter (Discrete or Continuous)1/1
  MATLAB Function/1(x_hat) -> sig_hat/1
  Low-Pass Filter (Discrete or Continuous)/1 -> MATLAB Function/2(z2)
  sig1/1 -> Low-Pass Filter (Discrete or Continuous)2/1
  sig2/1 -> Low-Pass Filter (Discrete or Continuous)/1
  Low-Pass Filter (Discrete or Continuous)2/1 -> MATLAB Function/1(z1)
  Low-Pass Filter (Discrete or Continuous)1/1 -> MATLAB Function/3(z3)

== system VELO1/Subsystem/StateTransition ==
  stateTransitionFcn : TriggerPort  TriggerType=function-call  IsSimulinkFunction=on  FunctionName=stateTransitionFcn  FunctionVisibility=scoped  VariantControl=(inherit)
  Add : Sum
  x : ArgIn  DisableCoverage=on  ArgumentName=x
  w : ArgIn  Port=2  ArgumentName=w
  xNext : ArgOut  DisableCoverage=on  ArgumentName=xNext
  wires:
  w/1 -> Add/2
  Add/1 -> xNext/1
  x/1 -> Add/1

== system VELO1/Subsystem/sig1 Measurement ==
  Temp1MeasurementFcn : TriggerPort  TriggerType=function-call  IsSimulinkFunction=on  FunctionName=sig1MeasurementFcn  FunctionVisibility=scoped  VariantControl=(inherit)
  Add : Sum  Inputs=+++
  Constant : Constant
  x : ArgIn  DisableCoverage=on  ArgumentName=x
  v : ArgIn  Port=2  ArgumentName=v
  y : ArgOut  DisableCoverage=on  ArgumentName=y
  wires:
  Add/1 -> y/1
  x/1 -> Add/1  "state"
  Constant/1 -> Add/2  "bias"
  v/1 -> Add/3  "noise"

== system VELO1/Subsystem/sig2 Measurement ==
  sig2MeasurementFcn : TriggerPort  TriggerType=function-call  IsSimulinkFunction=on  FunctionName=sig2MeasurementFcn  FunctionVisibility=scoped  VariantControl=(inherit)
  Add : Sum  Inputs=+++
  Constant : Constant  Value=-1
  x : ArgIn  DisableCoverage=on  ArgumentName=x
  v : ArgIn  Port=2  ArgumentName=v
  y : ArgOut  DisableCoverage=on  ArgumentName=y
  wires:
  v/1 -> Add/3
  Add/1 -> y/1
  Constant/1 -> Add/2
  x/1 -> Add/1

== system VELO1/Subsystem/sig3 Measurement1 ==
  sig2MeasurementFcn : TriggerPort  TriggerType=function-call  IsSimulinkFunction=on  FunctionName=sig2MeasurementFcn  FunctionVisibility=scoped  VariantControl=(inherit)
  Add : Sum  Inputs=+++
  Constant : Constant  Value=-1
  x : ArgIn  DisableCoverage=on  ArgumentName=x
  v : ArgIn  Port=2  ArgumentName=v
  y : ArgOut  DisableCoverage=on  ArgumentName=y
  wires:
  x/1 -> Add/1
  Constant/1 -> Add/2
  Add/1 -> y/1
  v/1 -> Add/3

== system VELO1/speed/Subsystem ==
  Mux : Mux
  Scope10 : Scope
  To Workspace : ToWorkspace  VariableName=V_W  SaveFormat=Timeseries  SampleTime=-1
  wires:
  [V_w3] -> Mux/3
  [V_w2] -> Mux/2
  [V_w1] -> Mux/1
  Mux/1 -> Scope10/1, To Workspace/1
  [V_w4] -> Mux/4

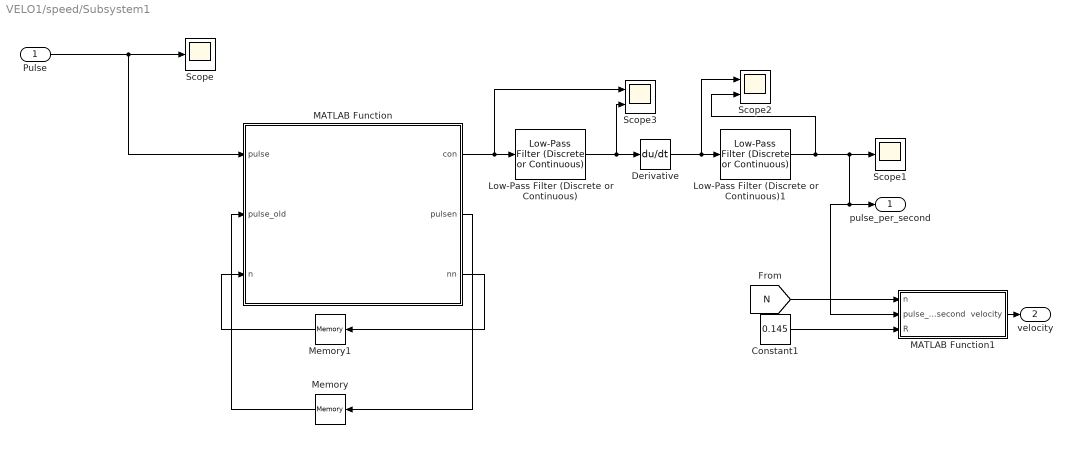
== system VELO1/speed/Subsystem1 ==
  Pulse : Inport
  Constant1 : Constant  Value=0.145
  Derivative : Derivative
  Low-Pass Filter (Discrete or Continuous) : eeGeneralControl/Low-Pass Filter (Discrete or Continuous)  K=1  T=0.4  B=inf  A=-inf  Ts=-1
      settings: SourceProductName=Simscape Electrical
  Low-Pass Filter (Discrete or Continuous)1 : eeGeneralControl/Low-Pass Filter (Discrete or Continuous)  K=1  T=0.2  B=inf  A=-inf  Ts=-1
      settings: SourceProductName=Simscape Electrical
  MATLAB Function : MATLAB Function  TreatAsAtomicUnit=on
  MATLAB Function1 : MATLAB Function  TreatAsAtomicUnit=on
  Memory : Memory
  Memory1 : Memory
  Scope : Scope
  Scope1 : Scope
  Scope2 : Scope  NumInputPorts=2
  Scope3 : Scope  NumInputPorts=2
  pulse_per_second : Outport
  velocity : Outport  Port=2
  wires:
  Low-Pass Filter (Discrete or Continuous)/1 -> Derivative/1, Scope3/2
  Derivative/1 -> Low-Pass Filter (Discrete or Continuous)1/1, Scope2/1
  Memory/1 -> MATLAB Function/2(pulse_old)
  Pulse/1 -> MATLAB Function/1(pulse), Scope/1
  MATLAB Function/2(pulsen) -> Memory/1
  MATLAB Function/3(nn) -> Memory1/1
  Memory1/1 -> MATLAB Function/3(n)
  MATLAB Function/1(con) -> Scope3/1, Low-Pass Filter (Discrete or Continuous)/1
  Low-Pass Filter (Discrete or Continuous)1/1 -> pulse_per_second/1, MATLAB Function1/2(pulse_per_second), Scope1/1, Scope2/2
  [N] -> MATLAB Function1/1(n)
  Constant1/1 -> MATLAB Function1/3(R)
  MATLAB Function1/1(velocity) -> velocity/1

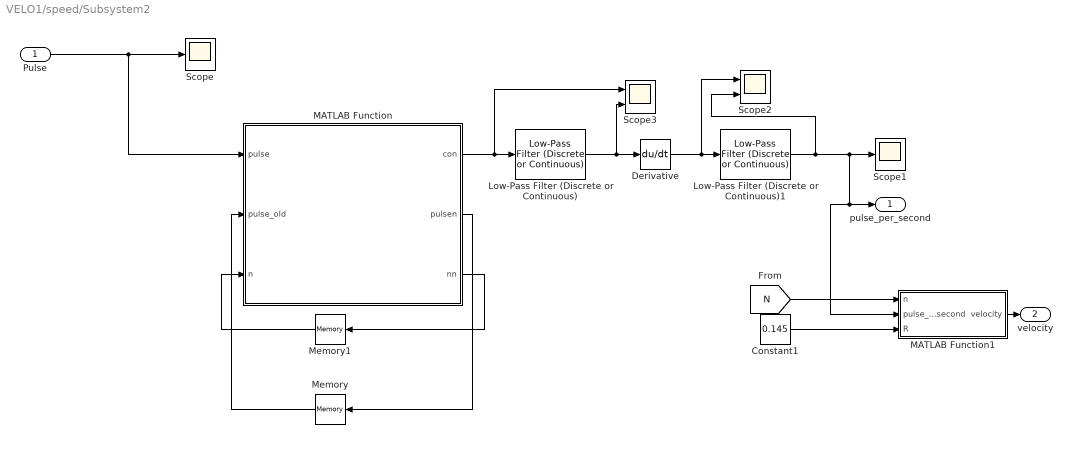
== system VELO1/speed/Subsystem2 ==
  Pulse : Inport
  Constant1 : Constant  Value=0.145
  Derivative : Derivative
  Low-Pass Filter (Discrete or Continuous) : eeGeneralControl/Low-Pass Filter (Discrete or Continuous)  K=1  T=0.4  B=inf  A=-inf  Ts=-1
      settings: SourceProductName=Simscape Electrical
  Low-Pass Filter (Discrete or Continuous)1 : eeGeneralControl/Low-Pass Filter (Discrete or Continuous)  K=1  T=0.2  B=inf  A=-inf  Ts=-1
      settings: SourceProductName=Simscape Electrical
  MATLAB Function : MATLAB Function  TreatAsAtomicUnit=on
  MATLAB Function1 : MATLAB Function  TreatAsAtomicUnit=on
  Memory : Memory
  Memory1 : Memory
  Scope : Scope
  Scope1 : Scope
  Scope2 : Scope  NumInputPorts=2
  Scope3 : Scope  NumInputPorts=2
  pulse_per_second : Outport
  velocity : Outport  Port=2
  wires:
  MATLAB Function1/1(velocity) -> velocity/1
  Constant1/1 -> MATLAB Function1/3(R)
  [N] -> MATLAB Function1/1(n)
  Low-Pass Filter (Discrete or Continuous)1/1 -> Scope2/2, Scope1/1, MATLAB Function1/2(pulse_per_second), pulse_per_second/1
  MATLAB Function/1(con) -> Low-Pass Filter (Discrete or Continuous)/1, Scope3/1
  Memory1/1 -> MATLAB Function/3(n)
  MATLAB Function/3(nn) -> Memory1/1
  MATLAB Function/2(pulsen) -> Memory/1
  Pulse/1 -> Scope/1, MATLAB Function/1(pulse)
  Memory/1 -> MATLAB Function/2(pulse_old)
  Derivative/1 -> Scope2/1, Low-Pass Filter (Discrete or Continuous)1/1
  Low-Pass Filter (Discrete or Continuous)/1 -> Scope3/2, Derivative/1

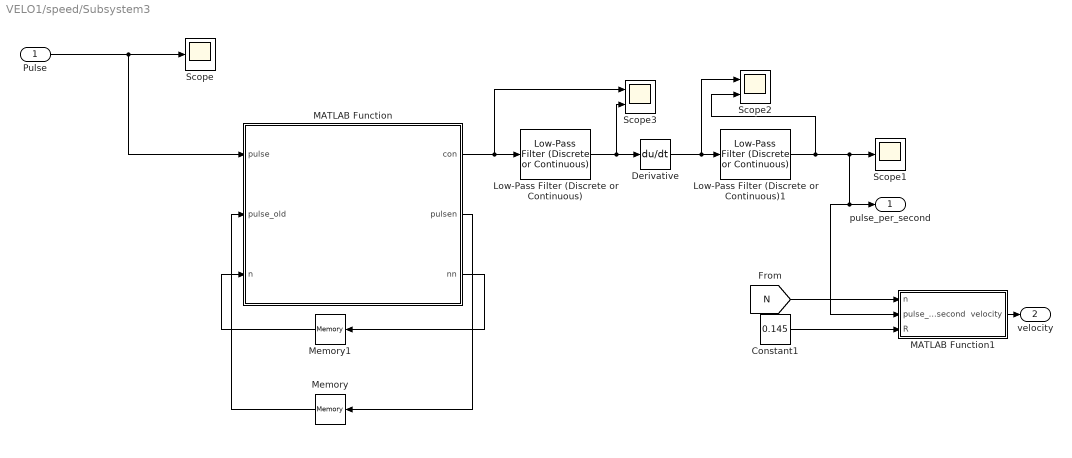
== system VELO1/speed/Subsystem3 ==
  Pulse : Inport
  Constant1 : Constant  Value=0.145
  Derivative : Derivative
  Low-Pass Filter (Discrete or Continuous) : eeGeneralControl/Low-Pass Filter (Discrete or Continuous)  K=1  T=0.4  B=inf  A=-inf  Ts=-1
      settings: SourceProductName=Simscape Electrical
  Low-Pass Filter (Discrete or Continuous)1 : eeGeneralControl/Low-Pass Filter (Discrete or Continuous)  K=1  T=0.2  B=inf  A=-inf  Ts=-1
      settings: SourceProductName=Simscape Electrical
  MATLAB Function : MATLAB Function  TreatAsAtomicUnit=on
  MATLAB Function1 : MATLAB Function  TreatAsAtomicUnit=on
  Memory : Memory
  Memory1 : Memory
  Scope : Scope
  Scope1 : Scope
  Scope2 : Scope  NumInputPorts=2
  Scope3 : Scope  NumInputPorts=2
  pulse_per_second : Outport
  velocity : Outport  Port=2
  wires:
  MATLAB Function1/1(velocity) -> velocity/1
  Constant1/1 -> MATLAB Function1/3(R)
  [N] -> MATLAB Function1/1(n)
  Low-Pass Filter (Discrete or Continuous)1/1 -> Scope2/2, Scope1/1, MATLAB Function1/2(pulse_per_second), pulse_per_second/1
  Memory1/1 -> MATLAB Function/3(n)
  MATLAB Function/3(nn) -> Memory1/1
  MATLAB Function/2(pulsen) -> Memory/1
  Pulse/1 -> Scope/1, MATLAB Function/1(pulse)
  Memory/1 -> MATLAB Function/2(pulse_old)
  Derivative/1 -> Scope2/1, Low-Pass Filter (Discrete or Continuous)1/1
  MATLAB Function/1(con) -> Low-Pass Filter (Discrete or Continuous)/1, Scope3/1
  Low-Pass Filter (Discrete or Continuous)/1 -> Scope3/2, Derivative/1

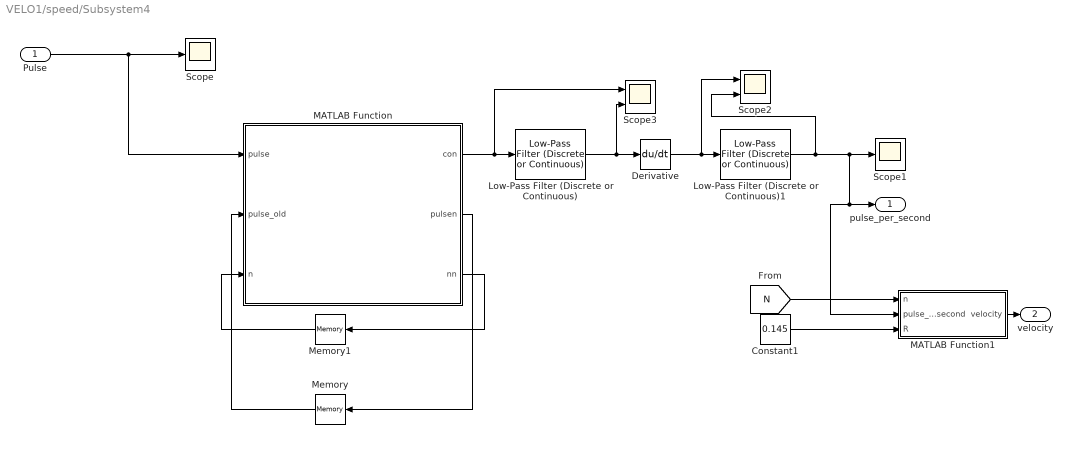
== system VELO1/speed/Subsystem4 ==
  Pulse : Inport
  Constant1 : Constant  Value=0.145
  Derivative : Derivative
  Low-Pass Filter (Discrete or Continuous) : eeGeneralControl/Low-Pass Filter (Discrete or Continuous)  K=1  T=0.4  B=inf  A=-inf  Ts=-1
      settings: SourceProductName=Simscape Electrical
  Low-Pass Filter (Discrete or Continuous)1 : eeGeneralControl/Low-Pass Filter (Discrete or Continuous)  K=1  T=0.2  B=inf  A=-inf  Ts=-1
      settings: SourceProductName=Simscape Electrical
  MATLAB Function : MATLAB Function  TreatAsAtomicUnit=on
  MATLAB Function1 : MATLAB Function  TreatAsAtomicUnit=on
  Memory : Memory
  Memory1 : Memory
  Scope : Scope
  Scope1 : Scope
  Scope2 : Scope  NumInputPorts=2
  Scope3 : Scope  NumInputPorts=2
  pulse_per_second : Outport
  velocity : Outport  Port=2
  wires:
  Low-Pass Filter (Discrete or Continuous)/1 -> Derivative/1, Scope3/2
  Derivative/1 -> Low-Pass Filter (Discrete or Continuous)1/1, Scope2/1
  Memory/1 -> MATLAB Function/2(pulse_old)
  Pulse/1 -> MATLAB Function/1(pulse), Scope/1
  MATLAB Function/2(pulsen) -> Memory/1
  MATLAB Function/3(nn) -> Memory1/1
  Memory1/1 -> MATLAB Function/3(n)
  MATLAB Function/1(con) -> Scope3/1, Low-Pass Filter (Discrete or Continuous)/1
  Low-Pass Filter (Discrete or Continuous)1/1 -> pulse_per_second/1, MATLAB Function1/2(pulse_per_second), Scope1/1, Scope2/2
  [N] -> MATLAB Function1/1(n)
  Constant1/1 -> MATLAB Function1/3(R)
  MATLAB Function1/1(velocity) -> velocity/1

== system VELO1/speed/Subsystem5 ==
  Moving Average{,1..3} (4 alike) : dspstat3/Moving Average  Method=Sliding window  ForgettingFactorPort=off  SpecifyWindowLength=on  WindowLength=50  ForgettingFactor=0.9  SimulateUsing=Code generation
  Mux : Mux
  Scope10 : Scope
  To Workspace : ToWorkspace  VariableName=V_Wp  SaveFormat=Timeseries  SampleTime=-1
  wires:
  [V_w4] -> Moving Average/1
  Mux/1 -> To Workspace/1, Scope10/1
  [V_w1] -> Moving Average3/1
  [V_w2] -> Moving Average2/1
  [V_w3] -> Moving Average1/1
  Moving Average/1 -> Mux/4  "v_w4"
  Moving Average1/1 -> Mux/3  "v_w3"
  Moving Average2/1 -> Mux/2  "v_w2"
  Moving Average3/1 -> Mux/1  "v_w1"

== matlab function VELO1/speed/Subsystem1/MATLAB Function ==
  data: pulse input; con output; pulse_old input; n input; pulsen output; nn output
function [con ,pulsen,nn] = fcn(pulse,pulse_old,n)

if pulse<pulse_old
    
    nn=n+1;
con=nn*255+pulse;

else 
 
con=n*255+pulse;
nn=n;
end
pulsen=pulse;
end

== matlab function VELO1/speed/Subsystem1/MATLAB Function1 ==
  data: n input; velocity output; pulse_per_second input; R input
function velocity = fcn(n,pulse_per_second,R)

velocity =(pulse_per_second*3.6/(2*pi*n))*R;
end

== matlab function VELO1/speed/Subsystem2/MATLAB Function ==
  data: pulse input; con output; pulse_old input; n input; pulsen output; nn output
function [con ,pulsen,nn] = fcn(pulse,pulse_old,n)

if pulse<pulse_old
    
    nn=n+1;
con=nn*255+pulse;

else 
 
con=n*255+pulse;
nn=n;
end
pulsen=pulse;
end

== matlab function VELO1/speed/Subsystem2/MATLAB Function1 ==
  data: n input; velocity output; pulse_per_second input; R input
function velocity = fcn(n,pulse_per_second,R)

velocity =(pulse_per_second*3.6/(2*pi*n))*R;
end

== matlab function VELO1/speed/Subsystem4/MATLAB Function ==
  data: pulse input; con output; pulse_old input; n input; pulsen output; nn output
function [con ,pulsen,nn] = fcn(pulse,pulse_old,n)

if pulse<pulse_old
    
    nn=n+1;
con=nn*255+pulse;

else 
 
con=n*255+pulse;
nn=n;
end
pulsen=pulse;
end

== matlab function VELO1/speed/Subsystem4/MATLAB Function1 ==
  data: n input; velocity output; pulse_per_second input; R input
function velocity = fcn(n,pulse_per_second,R)

velocity =(pulse_per_second*3.6/(2*pi*n))*R;
end

== matlab function VELO1/speed/Subsystem3/MATLAB Function ==
  data: pulse input; con output; pulse_old input; n input; pulsen output; nn output
function [con ,pulsen,nn] = fcn(pulse,pulse_old,n)

if pulse<pulse_old
    
    nn=n+1;
con=nn*255+pulse;

else 
 
con=n*255+pulse;
nn=n;
end
pulsen=pulse;
end

== matlab function VELO1/speed/Subsystem3/MATLAB Function1 ==
  data: n input; velocity output; pulse_per_second input; R input
function velocity = fcn(n,pulse_per_second,R)

velocity =(pulse_per_second*3.6/(2*pi*n))*R;
end

== matlab function VELO1/speed/MATLAB Function ==
  data: a input; D output; b input; c input; d input
function D = fcn(a,b,c,d)

D=(a*c)/(b*d);

end

== matlab function VELO1/Raw data filer /Subsystem1/MATLAB Function ==
  data: z1 input; x_hat output; z2 input; z3 input
function x_hat=fusion(z1,z2,z3)
% Kalman Filter sensor fusion example based on
%  
% http://www.slideshare.net/antoniomorancardenas/data-fusion-with-kalman-filtering
%
% % See http://home.wlu.edu/~levys/kalman_tutorial for background

% Copyright (C) 2014 Simon D. Levy
%
% This code is free software: you can redistribute it and/or modify
% it under the terms of the GNU Lesser General Public License as
% published by the Free Software Foundation, either version 3 of the
% License, or (at your option) any later version.
%
% This code is distributed in the hope that it will be useful,
% but WITHOUT ANY WARRANTY without even the implied warranty of
% MERCHANTABILITY or FITNESS FOR A PARTICULAR PURPOSE. See the
% GNU General Public License for more details.
%
% You should have received a copy of the GNU Lesser General Public License
% along with this code. If not, see <http:#www.gnu.org/licenses/>.

% Parameters ============================================================

% Biases
% BIAS1 = +1;
% BIAS2 = -1;

% Measurement noise covariances
R1 = 0.64;
R2 = 0.64;
R3 = 0.64;
% Process noise covariance
Q = .005;

% State transition model
A = 1;

% Observation model
C1 = 1;
C2 = 1;
C3=1;
% Duration
% N = 1000;

% Run ====================================================================

% Generate the signal x as a sine wave
% x = 20 + sin(5*linspace(0,1,N)*pi);

% Add some process noise with covariance Q
% w = sqrt(Q) * randn(size(x));
% x = x + w;

% Compute noisy sensor values
% z1 = BIAS1 + x + sqrt(R1) * randn(size(x));
% z2 = BIAS2 + x + sqrt(R2) * randn(size(x));

% Run a single-sensor example and plot it
% xhat = kalman(z1, A, C1, R1, Q);
% 
% % Plot sensed and estimated values
% clf
% plotsigs(1, z1, xhat, 'Sensor 1')
% title('One sensor: signal cleanup')
% 
% % Plot estimate and actual values
% plotsigsrms('One sensor', 2, x, xhat)

% Run the Kalman filter on fused sensors
x_hat = kalman([z1; z2; z3], A, [C1; C2 ;C3], [R1 0 0; 0 R2 0;0 0 R3], [Q;Q;Q]);
end

% Plot fusion example


% Helper functions ======================================================
